simulink model "hcu_main_ADASwEPS"  (Simulink 8.2)
settings: Solver=FixedStepDiscrete  StartTime=0.0  StopTime=inf  FixedStep=0.001  RelTol=1e-3
PostLoadFcn:
  | , if any(exist('dsrtsu_mdlpostloadfcn', 'file') == [2, 3, 6]), try dsrtsu_mdlpostloadfcn('Execute', bdroot); catch fprintf('Error in PostLoadFcn (dsrtsu_mdlpostloadfcn) for model "%s":\n %s\n', bdroot, lasterr); end, end,
values from neighbouring files (symbols this model uses):
  C_TASK_1MS_S = (	C_TICK_TIME_S       )    [hcu_local_hdr.m]    (also in temp_ovrd_values.m = double(	0.001                  ))
  C_TICK_TIME_S = single(	0.005	    	)    [hcu_local_hdr.m]
  ENUM_EPSLFCSTATUS_ACTIVE = uint8(  2  )    [hcu_local_hdr.m]
  ENUM_EPSLFCSTATUS_TRANSITION = uint8(  3  )    [hcu_local_hdr.m]
  ENUM_EPSLKASTATUS_ACTIVE = uint8(  2  )    [hcu_local_hdr.m]
  ENUM_EPSMODEREQ_ANGLE = uint8(  1  )    [hcu_local_hdr.m]
  ENUM_EPSMODEREQ_INTERNAL = uint8(  0  )    [hcu_local_hdr.m]
  ENUM_EPSMODEREQ_TORQUE = uint8(  2  )    [hcu_local_hdr.m]
  ENUM_GEARPOSN_1ST = uint8(  1  )    [hcu_local_hdr.m]
  ENUM_GEARPOSN_2ND = uint8(  2  )    [hcu_local_hdr.m]
  ENUM_GEARPOSN_3RD = uint8(  3  )    [hcu_local_hdr.m]
  ENUM_GEARPOSN_4TH = uint8(  4  )    [hcu_local_hdr.m]
  ENUM_GEARPOSN_5TH = uint8(  5  )    [hcu_local_hdr.m]
  ENUM_GEARPOSN_6TH = uint8(  6  )    [hcu_local_hdr.m]
  ENUM_GEARPOSN_R = uint8(  7  )    [hcu_local_hdr.m]
  FALSE = boolean( 0 )    [hcu_local_hdr.m]
  TRUE = boolean( 1 )    [hcu_local_hdr.m]
undefined symbols (not defined in the file or in its folder): AISP_EPSCurrent_pct, AISP_TqASensorDelta_pct, AISP_TqBSensorDelta_pct, dHAL_IN, hal, INVALID_ABS1_TIMEOUT, INVALID_ABS2_TIMEOUT, INVALID_ABS3_TIMEOUT, INVALID_ABS4_TIMEOUT, INVALID_AC1_TIMEOUT, INVALID_ADASTORQ_REQ, INVALID_BCM1_TIMEOUT, INVALID_BCM2_TIMEOUT, INVALID_BOOSTER_VAC, INVALID_CSW1_TIMEOUT, INVALID_CUR_VEHDECE, INVALID_CURBRAKEDECE_REQ, INVALID_CURSTEERANG_REQ, INVALID_CURSTEERTQ_REQ, INVALID_ECM1_TIMEOUT, INVALID_ECM2_TIMEOUT, INVALID_ECM3_TIMEOUT, INVALID_ECM9_TIMEOUT, INVALID_ENG_TORQUE_FRICTIONAL, INVALID_ENG_TORQUE_INDICATED, INVALID_ENG_TORQUE_INDICATEDCOR, INVALID_ENG_TQ_MAX, INVALID_ENG_TQ_MIN, INVALID_EPAS2_TIMEOUT, INVALID_EPAS3_TIMEOUT, INVALID_EPB1_TIMEOUT, INVALID_EPS_BATTVOLT, INVALID_ESC_BATTVOLT, INVALID_GRADE, INVALID_HCU3_TIMEOUT, INVALID_HCU4_TIMEOUT, INVALID_HMI1_TIMEOUT, INVALID_HMI2_TIMEOUT, INVALID_LAT_ACC, INVALID_LONG_ACC, INVALID_MC_PRESSURE, INVALID_METER1_TIMEOUT, INVALID_METER3_TIMEOUT, INVALID_METER_VEHSPD, INVALID_ODO_METER, INVALID_OUTSIDE_TEMP, INVALID_PARKBRAKEBIND_STAT, INVALID_PEDALTQ_REQ, INVALID_SAS1_TIMEOUT, INVALID_SAS_ANGLE, INVALID_SHIFTER_POSN, INVALID_TCM1_TIMEOUT, INVALID_TCM2_TIMEOUT, INVALID_VCU1_TIMEOUT, INVALID_VCU2_TIMEOUT, INVALID_VEH_CRASH, INVALID_VEH_SPD, INVALID_WHEEL_SPD, INVALID_YAW_RATE, KHAL_MssgIdObj1_num ... (+8)
libraries: simulink x147, hcu_lib x38, rti1401lib_dio_type3 x4, rtimmsu_dsrtlib x3, app x1, rtiethernetudplib x1, rti1401lib_adc_type4 x1, rti1401lib_dac_type3 x1, inp x1, lidr x1, outp x1
(part 8 of 15)

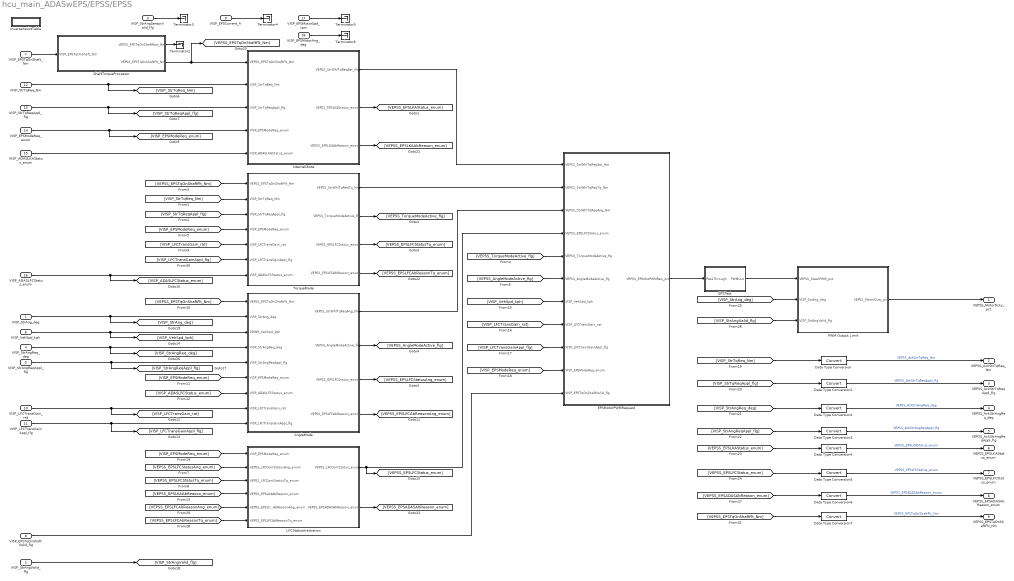
== system hcu_main_ADASwEPS/EPSS/EPSS ==
  VISP_StrAng_deg : Inport
  VISP_StrAngValid_flg : Inport  Port=2
  VISP_StrAngSensorValid_flg : Inport  Port=3
  VISP_StrAngReq_deg : Inport  Port=4
  VISP_StrAngReqAppl_flg : Inport  Port=5
  VISP_VehSpd_kph : Inport  Port=6
  VISP_EPSTqOnShaft_Nm : Inport  Port=7
  VISP_EPSTqOnShaftValid_flg : Inport  Port=8
  VISP_EPSCurrent_A : Inport  Port=9
  VISP_LFCTransGain_rat : Inport  Port=10
  VISP_LFCTransGainAppl_flg : Inport  Port=11
  VISP_StrTqReq_Nm : Inport  Port=12
  VISP_StrTqReqAppl_flg : Inport  Port=13
  VISP_EPSModeReq_enum : Inport  Port=14
  VISP_ADASLKAStatus_enum : Inport  Port=15
  VISP_ADASLFCStatus_enum : Inport  Port=16
  VISP_EPSMotorSpd_rpm : Inport  Port=17
  VISP_EPSMotorAng_deg : Inport  Port=18
  AngleMode : Subsystem
  Data Type Conversion{,1..7} (8 alike) : DataTypeConversion
  EPSMotorPWMRequest : Subsystem
  EPSTest : Subsystem
  InternalMode : Subsystem
  InverseAssistTable : Subsystem
  LFCStatusArbitration : Subsystem
  PWM Output Limit : Subsystem
  ShaftTorqueProcessor : Subsystem
  Terminator{2..6} (5 alike) : Terminator
  TorqueMode : Subsystem
  VEPSS_MotorDuty_pct : Outport
  VEPSS_AckStrTqReq_Nm : Outport  Port=2
  VEPSS_AckStrTqReqAppl_flg : Outport  Port=3
  VEPSS_AckStrAngReq_deg : Outport  Port=4
  VEPSS_AckStrAngReqAppl_flg : Outport  Port=5
  VEPSS_EPSLKAStatus_enum : Outport  Port=6
  VEPSS_EPSLFCStatus_enum : Outport  Port=7
  VEPSS_EPSADASAbReason_enum : Outport  Port=8
  VEPSS_EPSTqOnShaftFlt_Nm : Outport  Port=9
  wires:
  PWM Output Limit/1(VEPSS_MotorDuty_pct) -> VEPSS_MotorDuty_pct/1
  EPSMotorPWMRequest/1(VEPSS_EPSMotPWMReq_pct) -> EPSTest/1(PassThrough)
  EPSTest/1(PWMOut) -> PWM Output Limit/1(VEPSS_SteerPWM_pct)
  ShaftTorqueProcessor/2(VEPSS_EPSTqOnShaftFlt_Nm) -> [VEPSS_EPSTqOnShaftFlt_Nm], InternalMode/1(VEPSS_EPSTqOnShaftFlt_Nm)
  TorqueMode/1(VEPSS_StrWhlTqReqTq_Nm) -> EPSMotorPWMRequest/2(VEPSS_StrWhlTqReqTq_Nm)
  AngleMode/1(VEPSS_StrWhlTqReqAng_Nm) -> EPSMotorPWMRequest/3(VEPSS_StrWhlTqReqAng_Nm)
  InternalMode/1(VEPSS_StrWhlTqReqAst_Nm) -> EPSMotorPWMRequest/1(VEPSS_StrWhlTqReqAst_Nm)
  InternalMode/2(VEPSS_EPSLKAStatus_enum) -> [VEPSS_EPSLKAStatus_enum]
  TorqueMode/2(VEPSS_TorqueModeActive_flg) -> [VEPSS_TorqueModeActive_flg]
  TorqueMode/3(VEPSS_EPSLFCStatus_enum) -> [VEPSS_EPSLFCStatusTq_enum]
  AngleMode/2(VEPSS_AngleModeActive_flg) -> [VEPSS_AngleModeActive_flg]
  AngleMode/3(VEPSS_EPSLFCStatus_enum) -> [VEPSS_EPSLFCStatusAng_enum]
  [VEPSS_TorqueModeActive_flg] -> EPSMotorPWMRequest/5(VEPSS_TorqueModeActive_flg)
  [VEPSS_AngleModeActive_flg] -> EPSMotorPWMRequest/6(VEPSS_AngleModeActive_flg)
  LFCStatusArbitration/1(VEPSS_LFCContStatus_enum) -> EPSMotorPWMRequest/4(VEPSS_EPSLFCStatus_enum), [VEPSS_EPSLFCStatus_enum]
  [VEPSS_EPSLFCStatusTq_enum] -> LFCStatusArbitration/3(VEPSS_LFCContStatusTq_enum)
  [VEPSS_EPSLFCStatusAng_enum] -> LFCStatusArbitration/2(VEPSS_LFCContStatusAng_enum)
  ShaftTorqueProcessor/1(VEPSS_EPSTqOnShaftRaw_Nm) -> Terminator2/1
  VISP_EPSTqOnShaft_Nm/1 -> ShaftTorqueProcessor/1(VISP_EPSTqOnShaft_Nm)
  VISP_StrTqReqAppl_flg/1 -> [VISP_StrTqReqAppl_flg], InternalMode/3(VISP_StrTqReqAppl_flg)
  VISP_StrTqReq_Nm/1 -> [VISP_StrTqReq_Nm], InternalMode/2(VISP_StrTqReq_Nm)
  VISP_EPSModeReq_enum/1 -> [VISP_EPSModeReq_enum], InternalMode/4(VISP_EPSModeReq_enum)
  VISP_ADASLKAStatus_enum/1 -> InternalMode/5(VISP_ADASLKAStatus_enum)
  [VISP_StrTqReq_Nm] -> TorqueMode/2(VISP_StrTqReq_Nm)
  [VISP_StrTqReqAppl_flg] -> TorqueMode/3(VISP_StrTqReqAppl_flg)
  [VEPSS_EPSTqOnShaftFlt_Nm] -> TorqueMode/1(VEPSS_EPSTqOnShaftFlt_Nm)
  [VISP_EPSModeReq_enum] -> TorqueMode/4(VISP_EPSModeReq_enum)
  VISP_ADASLFCStatus_enum/1 -> [VISP_ADASLFCStatus_enum], TorqueMode/7(VISP_ADASLFCStatus_enum)
  VISP_StrAng_deg/1 -> [VISP_StrAng_deg], AngleMode/2(VISP_StrAng_deg)
  VISP_StrAngReq_deg/1 -> [VISP_StrAngReq_deg], AngleMode/4(VISP_StrAngReq_deg)
  VISP_StrAngReqAppl_flg/1 -> [VISP_StrAngReqAppl_flg], AngleMode/5(VISP_StrAngReqAppl_flg)
  [VEPSS_EPSTqOnShaftFlt_Nm] -> AngleMode/1(VEPSS_EPSTqOnShaftFlt_Nm)
  [VISP_EPSModeReq_enum] -> AngleMode/6(VISP_EPSModeReq_enum)
  [VISP_ADASLFCStatus_enum] -> AngleMode/7(VISP_ADASLFCStatus_enum)
  VISP_LFCTransGain_rat/1 -> [VISP_LFCTransGain_rat], AngleMode/8(VISP_LFCTransGain_rat)
  VISP_LFCTransGainAppl_flg/1 -> [VISP_LFCTransGainAppl_flg], AngleMode/9(VISP_LFCTransGainAppl_flg)
  [VISP_EPSModeReq_enum] -> LFCStatusArbitration/1(VISP_EPSModeReq_enum)
  VISP_VehSpd_kph/1 -> [VISP_VehSpd_kph], AngleMode/3(VDINR_VehSpd_kph)
  [VISP_VehSpd_kph] -> EPSMotorPWMRequest/7(VISP_VehSpd_kph)
  [VISP_LFCTransGain_rat] -> EPSMotorPWMRequest/8(VISP_LFCTransGain_rat)
  [VISP_LFCTransGainAppl_flg] -> EPSMotorPWMRequest/9(VISP_LFCTransGainAppl_flg)
  [VISP_EPSModeReq_enum] -> EPSMotorPWMRequest/10(VISP_EPSModeReq_enum)
  VISP_EPSTqOnShaftValid_flg/1 -> EPSMotorPWMRequest/11(VISP_EPSTqOnShaftValid_flg)
  VISP_StrAngValid_flg/1 -> [VISP_StrAngValid_flg]
  VISP_StrAngSensorValid_flg/1 -> Terminator3/1
  VISP_EPSCurrent_A/1 -> Terminator4/1
  VISP_EPSMotorSpd_rpm/1 -> Terminator5/1
  VISP_EPSMotorAng_deg/1 -> Terminator6/1
  [VISP_StrTqReqAppl_flg] -> Data Type Conversion1/1
  [VISP_StrAngReqAppl_flg] -> Data Type Conversion3/1
  [VEPSS_EPSLKAStatus_enum] -> Data Type Conversion4/1
  [VEPSS_EPSLFCStatus_enum] -> Data Type Conversion5/1
  Data Type Conversion/1 -> VEPSS_AckStrTqReq_Nm/1  "VEPSS_AckStrTqReq_Nm"
  Data Type Conversion1/1 -> VEPSS_AckStrTqReqAppl_flg/1  "VEPSS_AckStrTqReqAppl_flg"
  Data Type Conversion2/1 -> VEPSS_AckStrAngReq_deg/1  "VEPSS_AckStrAngReq_deg"
  Data Type Conversion3/1 -> VEPSS_AckStrAngReqAppl_flg/1  "VEPSS_AckStrAngReqAppl_flg"
  Data Type Conversion4/1 -> VEPSS_EPSLKAStatus_enum/1  "VEPSS_EPSLKAStatus_enum"
  Data Type Conversion5/1 -> VEPSS_EPSLFCStatus_enum/1  "VEPSS_EPSLFCStatus_enum"
  Data Type Conversion6/1 -> VEPSS_EPSADASAbReason_enum/1  "VEPSS_EPSADASAbReason_enum"
  [VISP_StrAng_deg] -> PWM Output Limit/2(VISP_StrAng_deg)
  [VISP_StrAngValid_flg] -> PWM Output Limit/3(VISP_StrAngValid_flg)
  InternalMode/3(VEPSS_EPSLKAAbReason_enum) -> [VEPSS_EPSLKAAbReason_enum]
  [VISP_LFCTransGain_rat] -> TorqueMode/5(VISP_LFCTransGain_rat)
  TorqueMode/4(VEPSS_EPSLFCAbReason_enum) -> [VEPSS_EPSLFCAbReasonTq_enum]
  AngleMode/4(VEPSS_EPSLFCAbReason_enum) -> [VEPSS_EPSLFCAbReasonAng_enum]
  [VEPSS_EPSLFCAbReasonAng_enum] -> LFCStatusArbitration/5(VEPSS_EPSLFCAbReasonAng_enum)
  [VEPSS_EPSLFCAbReasonTq_enum] -> LFCStatusArbitration/6(VEPSS_EPSLFCAbReasonTq_enum)
  LFCStatusArbitration/2(VEPSS_EPSADASAbReason_enum) -> [VEPSS_EPSADASAbReason_enum]
  [VEPSS_EPSADASAbReason_enum] -> Data Type Conversion6/1
  [VEPSS_EPSLKAAbReason_enum] -> LFCStatusArbitration/4(VEPSS_EPSLKAAbReason_enum)
  [VISP_StrTqReq_Nm] -> Data Type Conversion/1
  [VISP_StrAngReq_deg] -> Data Type Conversion2/1
  [VISP_LFCTransGainAppl_flg] -> TorqueMode/6(VISP_LFCTransGainAppl_flg)
  Data Type Conversion7/1 -> VEPSS_EPSTqOnShaftFlt_Nm/1  "VEPSS_EPSTqOnShaftFlt_Nm"
  [VEPSS_EPSTqOnShaftFlt_Nm] -> Data Type Conversion7/1

== system hcu_main_ADASwEPS/EPSS/model_info ==
  EmptySubsystem : Subsystem

== system hcu_main_ADASwEPS/ISP/AngleProcessing ==
  KISP_EPSZeroReset_flg : Inport
  VHAL_RelStrAng_deg : Inport  Port=2
  VHAL_VehSpd_kph : Inport  Port=3
  VHAL_YawRate_degps : Inport  Port=4
  VHAL_YawRateValid_flg : Inport  Port=5
  VHAL_LRRawWhlSpd_kph : Inport  Port=6
  VHAL_LRRawWhlSpdValid_flg : Inport  Port=7
  VHAL_RRRawWhlSpd_kph : Inport  Port=8
  VHAL_RRRawWhlSpdValid_flg : Inport  Port=9
  Abs : Abs
  Abs1 : Abs
  AbsAngCheckTime_s : Constant  Value=5
  Add : Sum  Inputs=+-
  Add1 : Sum  Inputs=+-
  KISP_AbsAngVehSpdthr_kph : Constant  Value=8
  KISP_AbsAngWhlSpdDifstr_kph : Constant  Value=0.5
  KISP_AbsAngYawRatethr_degps : Constant  Value=0.6
  Logical Operator : Logic  AllPortsSameDT=off  OutDataTypeStr=boolean
  Logical Operator1 : Logic  Operator=NOT  AllPortsSameDT=off  OutDataTypeStr=boolean
  Logical Operator2 : Logic  Inputs=6  AllPortsSameDT=off  OutDataTypeStr=boolean
  Logical Operator3 : Logic  Operator=OR  AllPortsSameDT=off  OutDataTypeStr=boolean
  Relational Operator : RelationalOperator  OutDataTypeStr=boolean
  Relational Operator1 : RelationalOperator  Operator=<=  OutDataTypeStr=boolean
  Relational Operator2 : RelationalOperator  OutDataTypeStr=boolean
  Relational Operator3 : RelationalOperator  Operator=<=  OutDataTypeStr=boolean
  Saturation : Saturate  UpperLimit=720  LowerLimit=-720
  Timer : Subsystem
  Triggered Absolute Angle Zero : Subsystem  TreatAsAtomicUnit=on
  Unit Delay : UnitDelay  SampleTime=-1
  VISP_StrAng_deg : Outport
  VISP_StrAngValid_flg : Outport  Port=2
  wires:
  VHAL_VehSpd_kph/1 -> Relational Operator/1
  KISP_AbsAngVehSpdthr_kph/1 -> Relational Operator/2
  VHAL_YawRate_degps/1 -> Abs/1
  Abs/1 -> Relational Operator1/1
  KISP_AbsAngYawRatethr_degps/1 -> Relational Operator1/2
  Relational Operator1/1 -> Timer/Enable
  Timer/1(Time_s) -> Relational Operator2/1
  AbsAngCheckTime_s/1 -> Relational Operator2/2
  VHAL_RRRawWhlSpd_kph/1 -> Add/2
  VHAL_LRRawWhlSpd_kph/1 -> Add/1
  Add/1 -> Abs1/1
  Abs1/1 -> Relational Operator3/1
  KISP_AbsAngWhlSpdDifstr_kph/1 -> Relational Operator3/2
  Relational Operator/1 -> Logical Operator2/1
  Relational Operator2/1 -> Logical Operator2/2
  VHAL_YawRateValid_flg/1 -> Logical Operator2/3
  VHAL_LRRawWhlSpdValid_flg/1 -> Logical Operator2/4
  Relational Operator3/1 -> Logical Operator2/5
  VHAL_RRRawWhlSpdValid_flg/1 -> Logical Operator2/6
  Logical Operator2/1 -> Logical Operator/1
  Unit Delay/1 -> Logical Operator1/1
  Triggered Absolute Angle Zero/2(Out2) -> VISP_StrAngValid_flg/1, Unit Delay/1  "VISP_StrAngValid_flg"
  Logical Operator1/1 -> Logical Operator/2
  Logical Operator/1 -> Logical Operator3/2
  VHAL_RelStrAng_deg/1 -> Add1/1, Triggered Absolute Angle Zero/1(In)
  Triggered Absolute Angle Zero/1(Out1) -> Add1/2
  Add1/1 -> Saturation/1
  Saturation/1 -> VISP_StrAng_deg/1  "VISP_StrAng_deg"
  Logical Operator3/1 -> Triggered Absolute Angle Zero/Trigger
  KISP_EPSZeroReset_flg/1 -> Logical Operator3/1

== system hcu_main_ADASwEPS/ISP/PassThrough ==
  VHAL_RelStrAng_deg : Inport
  VHAL_VehSpd_kph : Inport  Port=2
  VHAL_StrAngReqAppl_flg : Inport  Port=3
  VHAL_StrAngReq_deg : Inport  Port=4
  VHAL_LFCTransGainAppl_flg : Inport  Port=5
  VHAL_LFCTransGain_rat : Inport  Port=6
  VHAL_LatAccel_mps2 : Inport  Port=7
  VHAL_StrTqReqAppl_flg : Inport  Port=8
  VHAL_StrTqReq_Nm : Inport  Port=9
  VHAL_EPSModeReq_enum : Inport  Port=10
  VHAL_ADASLKAStatus_enum : Inport  Port=11
  VHAL_ADASLFCStatus_enum : Inport  Port=12
  VHAL_EPSMotorSpd_rpm : Inport  Port=13
  VHAL_EPSMotorAng_deg : Inport  Port=14
  Data Type Conversion{,1..12,14} (14 alike) : DataTypeConversion
  EPSDegTest : Subsystem
  SteerAngSensorValid : Constant  Value=TRUE
  StrAngCmdOvr : Constant  Value=FALSE
  StrAngCmdVal : Constant  Value=0
  Switch1 : Switch  Criteria=u2 ~= 0
  Switch2 : Switch  Criteria=u2 ~= 0
  VISP_StrAngSensorValid_flg : Outport
  VISP_StrAngReqAppl_flg : Outport  Port=2
  VISP_StrAngReq_deg : Outport  Port=3
  VISP_VehSpd_kph : Outport  Port=4
  VISP_RelStrAng_deg : Outport  Port=5
  VISP_LFCTransGainAppl_flg : Outport  Port=6
  VISP_LFCTransGain_rat : Outport  Port=7
  VISP_LatAccel_mps2 : Outport  Port=8
  VISP_StrTqReqAppl_flg : Outport  Port=9
  VISP_StrTqReq_Nm : Outport  Port=10
  VISP_EPSModeReq_enum : Outport  Port=11
  VISP_ADASLKAStatus_enum : Outport  Port=12
  VISP_ADASLFCStatus_enum : Outport  Port=13
  VISP_EPSMotorSpd_rpm : Outport  Port=14
  VISP_EPSMotorAng_deg : Outport  Port=15
  wires:
  SteerAngSensorValid/1 -> VISP_StrAngSensorValid_flg/1  "VISP_StrAngSensorValid_flg"
  VHAL_StrAngReqAppl_flg/1 -> Switch1/3
  Data Type Conversion/1 -> VISP_StrAngReq_deg/1  "VISP_StrAngReq_deg"
  Data Type Conversion1/1 -> VISP_StrAngReqAppl_flg/1  "VISP_StrAngReqAppl_flg"
  VHAL_VehSpd_kph/1 -> Data Type Conversion2/1
  Data Type Conversion2/1 -> VISP_VehSpd_kph/1  "VISP_VehSpd_kph"
  VHAL_RelStrAng_deg/1 -> Data Type Conversion3/1
  Data Type Conversion3/1 -> VISP_RelStrAng_deg/1  "VISP_RelStrAng_deg"
  StrAngCmdOvr/1 -> Switch1/1, Switch2/2, Switch1/2
  Switch1/1 -> Data Type Conversion1/1
  Switch2/1 -> Data Type Conversion/1
  StrAngCmdVal/1 -> EPSDegTest/1(PassThrough)
  EPSDegTest/1(DegOut) -> Switch2/1
  Data Type Conversion4/1 -> VISP_LFCTransGainAppl_flg/1  "VISP_LFCTransGainAppl_flg"
  Data Type Conversion5/1 -> VISP_LFCTransGain_rat/1  "VISP_LFCTransGain_rat"
  VHAL_LFCTransGainAppl_flg/1 -> Data Type Conversion4/1
  VHAL_LFCTransGain_rat/1 -> Data Type Conversion5/1
  VHAL_LatAccel_mps2/1 -> Data Type Conversion6/1
  Data Type Conversion6/1 -> VISP_LatAccel_mps2/1  "VISP_LatAccel_mps2"
  VHAL_StrTqReqAppl_flg/1 -> Data Type Conversion7/1
  Data Type Conversion7/1 -> VISP_StrTqReqAppl_flg/1  "VISP_StrTqReqAppl_flg"
  Data Type Conversion8/1 -> VISP_StrTqReq_Nm/1  "VISP_StrTqReq_Nm"
  VHAL_EPSMotorSpd_rpm/1 -> Data Type Conversion9/1
  Data Type Conversion9/1 -> VISP_EPSMotorSpd_rpm/1  "VISP_EPSMotorSpd_rpm"
  VHAL_EPSMotorAng_deg/1 -> Data Type Conversion10/1
  Data Type Conversion10/1 -> VISP_EPSMotorAng_deg/1  "VISP_EPSMotorAng_deg"
  VHAL_EPSModeReq_enum/1 -> Data Type Conversion11/1
  Data Type Conversion11/1 -> VISP_EPSModeReq_enum/1  "VISP_EPSModeReq_enum"
  VHAL_ADASLKAStatus_enum/1 -> Data Type Conversion12/1
  Data Type Conversion12/1 -> VISP_ADASLKAStatus_enum/1  "VISP_ADASLKAStatus_enum"
  VHAL_ADASLFCStatus_enum/1 -> Data Type Conversion14/1
  Data Type Conversion14/1 -> VISP_ADASLFCStatus_enum/1  "VISP_ADASLFCStatus_enum"
  VHAL_StrAngReq_deg/1 -> Switch2/3
  VHAL_StrTqReq_Nm/1 -> Data Type Conversion8/1

== system hcu_main_ADASwEPS/ISP/TqProcessing ==
  VHAL_TqSensorADuty_pct : Inport
  VHAL_TqSensorBDuty_pct : Inport  Port=2
  KISP_EPSZeroReset_flg : Inport  Port=3
  Add : Sum
  Gain : Gain  Gain=1/2
  LowPassFilter : Subsystem
  MISP_TqAOnShaft_Nm : Lookup  InputValues=AISP_TqASensorDelta_pct  Table=MISP_TqAOnShaft_Nm  LookUpMeth=Interpolation-Use End Values
      settings: AttributesFormatString="Input=\"%<InputValues>\"\\nOutput=\"%<Table>\""
  MISP_TqBOnShaft_Nm : Lookup  InputValues=AISP_TqBSensorDelta_pct  Table=MISP_TqBOnShaft_Nm  LookUpMeth=Interpolation-Use End Values
      settings: AttributesFormatString="Input=\"%<InputValues>\"\\nOutput=\"%<Table>\""
  Terminator5 : Terminator
  Terminator6 : Terminator
  TorqueValid : Subsystem
  TqSensorAZero : Subsystem
  TqSensorBZero : Subsystem
  TqSensorFlac_pct : Constant  Value=0.1
  VISP_EPSTqOnShaft_Nm : Outport
  VISP_EPSTqOnShaftValid_flg : Outport  Port=2
  wires:
  Gain/1 -> LowPassFilter/1(Raw)
  TqSensorBZero/2(delta) -> MISP_TqBOnShaft_Nm/1
  Add/1 -> Gain/1
  TqSensorAZero/2(delta) -> MISP_TqAOnShaft_Nm/1
  TqSensorAZero/1(zero) -> Terminator5/1
  TqSensorBZero/1(zero) -> Terminator6/1
  TqSensorFlac_pct/1 -> TqSensorBZero/2(TqSensorFlac_pct), TqSensorAZero/2(TqSensorFlac_pct)
  KISP_EPSZeroReset_flg/1 -> TqSensorBZero/3(KISP_EPSZeroReset_flg), TqSensorAZero/3(KISP_EPSZeroReset_flg)
  MISP_TqAOnShaft_Nm/1 -> TorqueValid/1(TqA), Add/1
  TorqueValid/1(TqValid_flg) -> VISP_EPSTqOnShaftValid_flg/1  "VISP_EPSTqOnShaftValid_flg"
  MISP_TqBOnShaft_Nm/1 -> TorqueValid/2(TqB), Add/2
  VHAL_TqSensorADuty_pct/1 -> TqSensorAZero/1(VHAL_TqSensorADuty_pct)
  VHAL_TqSensorBDuty_pct/1 -> TqSensorBZero/1(VHAL_TqSensorBDuty_pct)
  LowPassFilter/1(Out) -> VISP_EPSTqOnShaft_Nm/1  "VISP_EPSTqOnShaft_Nm"

== system hcu_main_ADASwEPS/OSP/OSP ==
  BISP_outputs : Inport
  BEPSS_outputs : Inport  Port=2
  Bus Creator5 : BusCreator  Inputs=24
  Bus Selector : BusSelector  OutputSignals=VEPSS_EPSTqOnShaftFlt_Nm
  Bus Selector1 : BusSelector  OutputSignals=VEPSS_MotorDuty_pct,VEPSS_AckStrAngReq_deg,VEPSS_AckStrTqReq_Nm,VEPSS_AckStrAngReqAppl_flg,VEPSS_AckStrTqReqAppl_flg,VEPSS_EPSLKAStatus_enum,VEPSS_EPSLFCStatus_enum,VEPSS_EPSADASAbReason_enum
  Bus Selector2 : BusSelector  OutputSignals=VISP_EPSTqOnShaftValid_flg
  Bus Selector3 : BusSelector  OutputSignals=VISP_StrAng_deg,VISP_RelStrAng_deg,VISP_StrAngValid_flg,VISP_StrAngSensorValid_flg
  CheckSum Calculation : Subsystem  TreatAsAtomicUnit=on
  CheckSum Calculation1 : Subsystem  TreatAsAtomicUnit=on
  CheckSum Calculation2 : Subsystem  TreatAsAtomicUnit=on
  Constant : Constant  Value=15  OutDataTypeStr=uint8
  Constant1 : Constant  Value=15  OutDataTypeStr=uint8
  Constant2 : Constant  Value=15  OutDataTypeStr=uint8
  Constant4 : Constant  Value=TRUE
  Constant5 : Constant  Value=0.01
  Constant6 : Constant  Value=0.01
  Constant7 : Constant  Value=0.01
  Data Type Conversion{1..2,7,11,17,23..24,33} (8 alike) : DataTypeConversion  OutDataTypeStr=double
  Data Type Conversion{4..5,10,16,18,25..26} (7 alike) : DataTypeConversion  OutDataTypeStr=boolean
  Data Type Conversion{3,15,19..22,27,29..30} (9 alike) : DataTypeConversion  OutDataTypeStr=uint8
  EPSBattVolt : Constant  Value=12
  EpasFailed : Constant  Value=FALSE
  Function Call Generator EPAS2 : Stateflow chart  TreatAsAtomicUnit=on
  Function Call Generator EPAS3 : Stateflow chart  TreatAsAtomicUnit=on
  Function Call Generator SAS1 : Stateflow chart  TreatAsAtomicUnit=on
  RollCnt : Subsystem
  RollCnt1 : Subsystem
  RollCnt2 : Subsystem
  ZeroPower : Constant  Value=0
  BOSP_outputs : Outport
  wires:
  Bus Creator5/1 -> BOSP_outputs/1
  EpasFailed/1 -> Data Type Conversion10/1
  Data Type Conversion10/1 -> Bus Creator5/9  "VOSP_EpasFailed_flg"
  Data Type Conversion11/1 -> Bus Creator5/8  "VOSP_ElectPWRConsumpt_A"
  Data Type Conversion1/1 -> Bus Creator5/14  "VOSP_MotorDuty_pct"
  BEPSS_outputs/1 -> [BEPSS_outputs], CheckSum Calculation2/1(BEPSS_outputs), Bus Selector1/1
  Bus Selector1/1 -> Data Type Conversion1/1  "<VEPSS_MotorDuty_pct>"
  BISP_outputs/1 -> Bus Selector2/1, CheckSum Calculation/1(BISP_outputs), CheckSum Calculation1/2(BISP_outputs), Bus Selector3/1
  Bus Selector3/1 -> Data Type Conversion2/1  "<VISP_StrAng_deg>"
  Data Type Conversion2/1 -> Bus Creator5/1  "VOSP_StrAng_deg"
  Data Type Conversion4/1 -> Bus Creator5/3  "VOSP_StrAngCal_flg"
  Data Type Conversion5/1 -> Bus Creator5/4  "VOSP_RelStrAngValid_flg"
  Bus Selector3/2 -> Data Type Conversion7/1  "<VISP_RelStrAng_deg>"
  Data Type Conversion7/1 -> Bus Creator5/2  "VOSP_RelStrAng_deg"
  Bus Selector3/4 -> Data Type Conversion16/1  "<VISP_StrAngSensorValid_flg>"
  Data Type Conversion16/1 -> Bus Creator5/5  "VOSP_StrAngSensorValid_flg"
  Bus Selector/1 -> Data Type Conversion17/1  "<VEPSS_EPSTqOnShaftFlt_Nm>"
  Data Type Conversion17/1 -> Bus Creator5/6  "VOSP_StrTq_Nm"
  Bus Selector2/1 -> Data Type Conversion18/1  "<VISP_EPSTqOnShaftValid_flg>"
  Data Type Conversion18/1 -> Bus Creator5/7  "VOSP_StrTqValid_flg"
  ZeroPower/1 -> Data Type Conversion11/1
  Constant/1 -> RollCnt/1(max)
  RollCnt/1(out) -> Data Type Conversion15/1, CheckSum Calculation/2(LifeCount)
  Constant1/1 -> RollCnt1/1(max)
  RollCnt1/1(out) -> Data Type Conversion19/1, CheckSum Calculation1/3(LifeCount)
  Data Type Conversion15/1 -> Bus Creator5/11  "VOSP_SAS1RollCnt_cnt"
  Data Type Conversion19/1 -> Bus Creator5/13  "VOSP_EPAS2RollCnt_cnt"
  Constant2/1 -> RollCnt2/1(max)
  RollCnt2/1(out) -> CheckSum Calculation2/2(LifeCount), Data Type Conversion20/1
  Data Type Conversion20/1 -> Bus Creator5/24  "VOSP_EPAS3RollCnt_cnt"
  CheckSum Calculation/1(VOSP_SAS1CalcChecksum_raw8) -> Data Type Conversion21/1
  Data Type Conversion21/1 -> Bus Creator5/10  "VOSP_SAS1CalcChecksum_raw8"
  Data Type Conversion22/1 -> Bus Creator5/12  "VOSP_EPAS2CalcChecksum_raw8"
  CheckSum Calculation1/1(VOSP_EPAS2CalcChecksum_raw8) -> Data Type Conversion22/1
  Bus Selector1/2 -> Data Type Conversion23/1  "<VEPSS_AckStrAngReq_deg>"
  Data Type Conversion23/1 -> Bus Creator5/15  "VOSP_AckStrAngReq_deg"
  Bus Selector1/3 -> Data Type Conversion24/1  "<VEPSS_AckStrTqReq_Nm>"
  Data Type Conversion24/1 -> Bus Creator5/16  "VOSP_AckStrTqReq_Nm"
  Bus Selector1/4 -> Data Type Conversion25/1  "<VEPSS_AckStrAngReqAppl_flg>"
  Data Type Conversion25/1 -> Bus Creator5/17  "VOSP_AckStrAngReqAppl_flg"
  Data Type Conversion26/1 -> Bus Creator5/18  "VOSP_AckStrTqReqAppl_flg"
  Bus Selector1/5 -> Data Type Conversion26/1  "<VEPSS_AckStrTqReqAppl_flg>"
  Bus Selector1/6 -> Data Type Conversion27/1  "<VEPSS_EPSLKAStatus_enum>"
  Data Type Conversion27/1 -> Bus Creator5/19  "VOSP_EPSLKAStatus_enum"
  Data Type Conversion29/1 -> Bus Creator5/21  "VOSP_EPSADASAbReason_enum"
  Bus Selector1/8 -> Data Type Conversion29/1  "<VEPSS_EPSADASAbReason_enum>"
  Data Type Conversion30/1 -> Bus Creator5/20  "VOSP_EPSLFCStatus_enum"
  Bus Selector1/7 -> Data Type Conversion30/1  "<VEPSS_EPSLFCStatus_enum>"
  Data Type Conversion33/1 -> Bus Creator5/22  "VOSP_EPSBattVolt_V"
  EPSBattVolt/1 -> Data Type Conversion33/1
  Bus Selector3/3 -> Data Type Conversion4/1  "<VISP_StrAngValid_flg>"
  Constant4/1 -> Data Type Conversion5/1
  Constant5/1 -> Function Call Generator SAS1/1(SampleTime_S)
  Function Call Generator SAS1/1(FunCall()) -> RollCnt/Trigger
  Constant6/1 -> Function Call Generator EPAS2/1(SampleTime_S)
  Function Call Generator EPAS2/1(FunCall()) -> RollCnt1/Trigger
  Constant7/1 -> Function Call Generator EPAS3/1(SampleTime_S)
  Function Call Generator EPAS3/1(FunCall()) -> RollCnt2/Trigger
  CheckSum Calculation2/1(VOSP_EPAS3CalcChecksum_raw8) -> Data Type Conversion3/1
  Data Type Conversion3/1 -> Bus Creator5/23  "VOSP_EPAS3CalcChecksum_raw8"
  [BEPSS_outputs] -> Bus Selector/1
  [BEPSS_outputs] -> CheckSum Calculation1/1(BEPSS_outputs)

== system hcu_main_ADASwEPS/RTI Data/RTI Data Store ==
  RTI Data Store : Subsystem  mask(RTI_DATA_STORE){}
      mask help:
      | RTI Data Store Block. This block is used by RTI to store internal model dependent data. Deleting this block will result in data loss.
      |
      | NEVER DELETE, COPY, OR MODIFY THIS BLOCK!
      mask Help:
      | RTI Data Store Block. This block is used by RTI to store internal model dependent data. Deleting this block will result in data loss.
      | 
      | NEVER DELETE, COPY, OR MODIFY THIS BLOCK!
      mask Display: text(0.5, 0.5, ' ', 'HorizontalAlignment', 'center');

== system hcu_main_ADASwEPS/RTICANMM ControllerSetup/ModelClose ==

== system hcu_main_ADASwEPS/RTICANMM ControllerSetup1/ModelClose ==

== system hcu_main_ADASwEPS/RTICANMM GeneralSetup/ModelClose ==

== system hcu_main_ADASwEPS/Triggering2CAN1/ADAS4 ==
  ADAS4_Kickout : Constant  Value=0
  buscreator : BusCreator  Inputs=1
  dt_ADAS4_Kickout : DataTypeConversion  RndMeth=Zero
  out : Outport
  wires:
  buscreator/1 -> out/1  "ADAS4"
  ADAS4_Kickout/1 -> dt_ADAS4_Kickout/1
  dt_ADAS4_Kickout/1 -> buscreator/1  "ADAS4_Kickout"

== system hcu_main_ADASwEPS/Triggering2CAN1/ADAS5 ==
  ADAS5_Kickout : Constant  Value=0
  buscreator : BusCreator  Inputs=1
  dt_ADAS5_Kickout : DataTypeConversion  RndMeth=Zero
  out : Outport
  wires:
  buscreator/1 -> out/1  "ADAS5"
  ADAS5_Kickout/1 -> dt_ADAS5_Kickout/1
  dt_ADAS5_Kickout/1 -> buscreator/1  "ADAS5_Kickout"

== system hcu_main_ADASwEPS/User2CAN1_/ADAS1 ==
  BOUTP_outputs : Inport  OutDataTypeStr=Bus: BOUTP_outputs
  ADAS1_Checksum : Ground
  Bus Selector : BusSelector  OutputSignals=VOUTP_ADAS1RollCnt_cnt,VOUTP_StrTqAppl_flg,VOUTP_StrAngAppl_flg,VOUTP_LFCTransGainAppl_flg,VOUTP_EPSModeReq_enum,VOUTP_ADASLKAStatus_enum,VOUTP_ADASLFCStatus_enum,VOUTP_StrTqReq_Nm,VOUTP_LFCTransGain_rat,VOUTP_StrAngReq_deg
  Data Type Conversion{1..10} (10 alike) : DataTypeConversion
  buscreator : BusCreator  Inputs=11
  out : Outport
  wires:
  buscreator/1 -> out/1  "ADAS1"
  ADAS1_Checksum/1 -> buscreator/1  "ADAS1_Checksum"
  Data Type Conversion2/1 -> buscreator/2  "ADAS1_LifeCount"
  Data Type Conversion1/1 -> buscreator/3  "ADAS_StrTqReq_A"
  Data Type Conversion3/1 -> buscreator/4  "ADAS_StrAngReq_A"
  Data Type Conversion5/1 -> buscreator/5  "ADAS_LFCTranGain_A"
  Data Type Conversion4/1 -> buscreator/6  "ADAS_EPSMode"
  Data Type Conversion6/1 -> buscreator/7  "ADAS_LKAStatus"
  Data Type Conversion8/1 -> buscreator/8  "ADAS_LFCStatus"
  Data Type Conversion7/1 -> buscreator/9  "ADAS_StrTqReq"
  Data Type Conversion9/1 -> buscreator/10  "ADAS_LFCTransGain"
  Data Type Conversion10/1 -> buscreator/11  "ADAS_StrAngReq"
  BOUTP_outputs/1 -> Bus Selector/1
  Bus Selector/2 -> Data Type Conversion1/1  "<VOUTP_StrTqAppl_flg>"
  Bus Selector/1 -> Data Type Conversion2/1  "<VOUTP_ADAS1RollCnt_cnt>"
  Bus Selector/3 -> Data Type Conversion3/1  "<VOUTP_StrAngAppl_flg>"
  Bus Selector/4 -> Data Type Conversion5/1  "<VOUTP_LFCTransGainAppl_flg>"
  Bus Selector/5 -> Data Type Conversion4/1  "<VOUTP_EPSModeReq_enum>"
  Bus Selector/6 -> Data Type Conversion6/1  "<VOUTP_ADASLKAStatus_enum>"
  Bus Selector/7 -> Data Type Conversion8/1  "<VOUTP_ADASLFCStatus_enum>"
  Bus Selector/8 -> Data Type Conversion7/1  "<VOUTP_StrTqReq_Nm>"
  Bus Selector/9 -> Data Type Conversion9/1  "<VOUTP_LFCTransGain_rat>"
  Bus Selector/10 -> Data Type Conversion10/1  "<VOUTP_StrAngReq_deg>"

== system hcu_main_ADASwEPS/User2CAN1_/ADAS2 ==
  BOUTP_outputs : Inport  OutDataTypeStr=Bus: BOUTP_outputs
  ADAS2_Checksum : Ground
  Bus Selector : BusSelector  OutputSignals=VOUTP_ADAS2RollCnt_cnt,VOUTP_VirtualGearRatio_enum,VOUTP_ADASACCStatus_enum,VOUTP_BrakeHapticReq_flg,VOUTP_VehHoldReq_flg,VOUTP_BrakePrefillReqAppl_flg,VOUTP_BrakePrefillReq_flg,VOUTP_AEBReqAppl_flg,VOUTP_AEBReq_flg,VOUTP_DecReq_mps2,VOUTP_ForceIdleAppl_flg,VOUTP_DecReqAppl_flg,VOUTP_PTTqReqAppl_flg,VOUTP_ForceIdle_flg,VOUTP_PTTqReq_Nm
  Data Type Conversion{1..11,13..16} (15 alike) : DataTypeConversion
  buscreator : BusCreator  Inputs=16
  out : Outport
  wires:
  buscreator/1 -> out/1  "ADAS2"
  ADAS2_Checksum/1 -> buscreator/1  "ADAS2_Checksum"
  Data Type Conversion2/1 -> buscreator/2  "ADAS2_LifeCount"
  Data Type Conversion1/1 -> buscreator/3  "ADAS_VirtualGear"
  Data Type Conversion3/1 -> buscreator/4  "ADAS_ACCStatus"
  Data Type Conversion5/1 -> buscreator/5  "ADAS_BHapticReq"
  Data Type Conversion4/1 -> buscreator/6  "ADAS_VehHoldReq"
  Data Type Conversion6/1 -> buscreator/7  "ADAS_BPrefillReq_A"
  Data Type Conversion8/1 -> buscreator/8  "ADAS_BPrefillReq"
  Data Type Conversion7/1 -> buscreator/9  "ADAS_AEBReq_A"
  Data Type Conversion9/1 -> buscreator/10  "ADAS_AEBReq"
  Data Type Conversion10/1 -> buscreator/11  "ADAS_DecReq"
  Data Type Conversion13/1 -> buscreator/12  "ADAS_ForceIdle_A"
  Data Type Conversion11/1 -> buscreator/13  "ADAS_DecReq_A"
  Data Type Conversion14/1 -> buscreator/14  "ADAS_PTTqReq_A"
  Data Type Conversion16/1 -> buscreator/15  "ADAS_ForceIdle"
  Data Type Conversion15/1 -> buscreator/16  "ADAS_PTTqReq"
  BOUTP_outputs/1 -> Bus Selector/1
  Bus Selector/1 -> Data Type Conversion2/1  "<VOUTP_ADAS2RollCnt_cnt>"
  Bus Selector/2 -> Data Type Conversion1/1  "<VOUTP_VirtualGearRatio_enum>"
  Bus Selector/3 -> Data Type Conversion3/1  "<VOUTP_ADASACCStatus_enum>"
  Bus Selector/4 -> Data Type Conversion5/1  "<VOUTP_BrakeHapticReq_flg>"
  Bus Selector/5 -> Data Type Conversion4/1  "<VOUTP_VehHoldReq_flg>"
  Bus Selector/6 -> Data Type Conversion6/1  "<VOUTP_BrakePrefillReqAppl_flg>"
  Bus Selector/7 -> Data Type Conversion8/1  "<VOUTP_BrakePrefillReq_flg>"
  Bus Selector/8 -> Data Type Conversion7/1  "<VOUTP_AEBReqAppl_flg>"
  Bus Selector/9 -> Data Type Conversion9/1  "<VOUTP_AEBReq_flg>"
  Bus Selector/10 -> Data Type Conversion10/1  "<VOUTP_DecReq_mps2>"
  Bus Selector/11 -> Data Type Conversion13/1  "<VOUTP_ForceIdleAppl_flg>"
  Bus Selector/12 -> Data Type Conversion11/1  "<VOUTP_DecReqAppl_flg>"
  Bus Selector/13 -> Data Type Conversion14/1  "<VOUTP_PTTqReqAppl_flg>"
  Bus Selector/14 -> Data Type Conversion16/1  "<VOUTP_ForceIdle_flg>"
  Bus Selector/15 -> Data Type Conversion15/1  "<VOUTP_PTTqReq_Nm>"

== system hcu_main_ADASwEPS/User2CAN1_/ADAS3 ==
  BOUTP_outputs : Inport  OutDataTypeStr=Bus: BOUTP_outputs
  ADAS3_Checksum : Ground
  Bus Selector : BusSelector  OutputSignals=VOUTP_ADAS3RollCnt_cnt,VOUTP_ShiftPosnReqAppl_flg,VOUTP_ShiftPosnReq_enum,VOUTP_VehSpdLimAppl_flg,VOUTP_GearPosnReqAppl_flg,VOUTP_GearPosnReq_enum,VOUTP_VehSpdLim_kph
  Data Type Conversion{7,9..11,13..14,16} (7 alike) : DataTypeConversion
  buscreator : BusCreator  Inputs=8
  out : Outport
  wires:
  buscreator/1 -> out/1  "ADAS3"
  ADAS3_Checksum/1 -> buscreator/1  "ADAS3_Checksum"
  Data Type Conversion7/1 -> buscreator/2  "ADAS3_LifeCount"
  Data Type Conversion9/1 -> buscreator/3  "ADAS_ShftPosnReq_A"
  Data Type Conversion10/1 -> buscreator/4  "ADAS_ShftPosnReq"
  Data Type Conversion13/1 -> buscreator/5  "ADAS_VehSpdLim_A"
  Data Type Conversion11/1 -> buscreator/6  "ADAS_GearPosnReq_A"
  Data Type Conversion14/1 -> buscreator/7  "ADAS_GearPosnReq"
  Data Type Conversion16/1 -> buscreator/8  "ADAS_VehSpdLim"
  BOUTP_outputs/1 -> Bus Selector/1
  Bus Selector/3 -> Data Type Conversion10/1  "<VOUTP_ShiftPosnReq_enum>"
  Bus Selector/4 -> Data Type Conversion13/1  "<VOUTP_VehSpdLimAppl_flg>"
  Bus Selector/2 -> Data Type Conversion9/1  "<VOUTP_ShiftPosnReqAppl_flg>"
  Bus Selector/5 -> Data Type Conversion11/1  "<VOUTP_GearPosnReqAppl_flg>"
  Bus Selector/1 -> Data Type Conversion7/1  "<VOUTP_ADAS3RollCnt_cnt>"
  Bus Selector/6 -> Data Type Conversion14/1  "<VOUTP_GearPosnReq_enum>"
  Bus Selector/7 -> Data Type Conversion16/1  "<VOUTP_VehSpdLim_kph>"

== system hcu_main_ADASwEPS/User2CAN1_/ADAS4 ==
  BOUTP_outputs : Inport  OutDataTypeStr=Bus: BOUTP_outputs
  Bus Selector : BusSelector  OutputSignals=VOUTP_ADASMILReq_flg,VOUTP_FaultWarningReq_flg,VOUTP_ForceLowBeam_flg,VOUTP_ADASFunOffSoundReq_flg,VOUTP_ADASFunOnSoundReq_flg,VOUTP_HazardWarningReq_flg,VOUTP_LFCHMIStatus_enum,VOUTP_LKAHMIStatus_enum,VOUTP_LFCWarningReq_flg,VOUTP_IGSAWarningReq_flg,VOUTP_AEBWarningReq_flg,VOUTP_ACCWarningReq_flg,VOUTP_FCWWarningReq_flg
  Data Type Conversion{1..30} (30 alike) : DataTypeConversion
  Ground{,1..9,12..16,19,21} (17 alike) : Ground
  buscreator : BusCreator  Inputs=30
  out : Outport
  wires:
  buscreator/1 -> out/1  "ADAS4"
  Data Type Conversion7/1 -> buscreator/1  "ADAS_MIL"
  Data Type Conversion9/1 -> buscreator/2  "ADASFaultWarnReq"
  Data Type Conversion10/1 -> buscreator/3  "ForceLowBeam"
  Data Type Conversion13/1 -> buscreator/6  "LeftTurnLightReq"
  Data Type Conversion11/1 -> buscreator/7  "RightTurnLightReq"
  Data Type Conversion14/1 -> buscreator/8  "HazardWarningReq"
  Data Type Conversion16/1 -> buscreator/9  "HapticWarningReq"
  Data Type Conversion6/1 -> buscreator/10  "APSEnable"
  Data Type Conversion8/1 -> buscreator/11  "PilotMode"
  Data Type Conversion1/1 -> buscreator/12  "IGSAStatus"
  Data Type Conversion3/1 -> buscreator/13  "LFCMode"
  Data Type Conversion2/1 -> buscreator/14  "MAPPStatus"
  Data Type Conversion4/1 -> buscreator/15  "MAPAStatus"
  Data Type Conversion5/1 -> buscreator/16  "LCSStatus"
  Data Type Conversion20/1 -> buscreator/17  "LFCStatus"
  Data Type Conversion21/1 -> buscreator/18  "LKAStatus"
  Data Type Conversion12/1 -> buscreator/19  "ACCStatus"
  Data Type Conversion17/1 -> buscreator/20  "FCWStatus"
  Data Type Conversion15/1 -> buscreator/21  "AEBStatus"
  Data Type Conversion18/1 -> buscreator/22  "MAPPHMIWarningReq"
  Data Type Conversion19/1 -> buscreator/23  "MAPAHMIWarningReq"
  Data Type Conversion27/1 -> buscreator/24  "LCSHMIWarningReq"
  Data Type Conversion28/1 -> buscreator/25  "LFCHMIWarningReq"
  Data Type Conversion22/1 -> buscreator/26  "LKAHMIWarningReq"
  Data Type Conversion24/1 -> buscreator/27  "IGSAHMIWarningReq"
  Data Type Conversion23/1 -> buscreator/28  "AEBHMIWarningReq"
  Data Type Conversion25/1 -> buscreator/29  "ACCHMIWarningReq"
  Data Type Conversion26/1 -> buscreator/30  "FCWHMIWarningReq"
  BOUTP_outputs/1 -> Bus Selector/1
  Bus Selector/1 -> Data Type Conversion7/1  "<VOUTP_ADASMILReq_flg>"
  Bus Selector/2 -> Data Type Conversion9/1  "<VOUTP_FaultWarningReq_flg>"
  Bus Selector/3 -> Data Type Conversion10/1  "<VOUTP_ForceLowBeam_flg>"
  Bus Selector/6 -> Data Type Conversion14/1  "<VOUTP_HazardWarningReq_flg>"
  Bus Selector/10 -> Data Type Conversion24/1  "<VOUTP_IGSAWarningReq_flg>"
  Bus Selector/11 -> Data Type Conversion23/1  "<VOUTP_AEBWarningReq_flg>"
  Bus Selector/12 -> Data Type Conversion25/1  "<VOUTP_ACCWarningReq_flg>"
  Bus Selector/13 -> Data Type Conversion26/1  "<VOUTP_FCWWarningReq_flg>"
  Ground/1 -> Data Type Conversion13/1
  Ground1/1 -> Data Type Conversion11/1
  Ground2/1 -> Data Type Conversion16/1
  Ground3/1 -> Data Type Conversion6/1
  Ground4/1 -> Data Type Conversion8/1
  Ground5/1 -> Data Type Conversion1/1
  Ground6/1 -> Data Type Conversion3/1
  Ground7/1 -> Data Type Conversion2/1
  Ground8/1 -> Data Type Conversion4/1
  Ground9/1 -> Data Type Conversion5/1
  Bus Selector/7 -> Data Type Conversion20/1  "<VOUTP_LFCHMIStatus_enum>"
  Bus Selector/8 -> Data Type Conversion21/1  "<VOUTP_LKAHMIStatus_enum>"
  Ground14/1 -> Data Type Conversion12/1
  Ground15/1 -> Data Type Conversion17/1
  Ground16/1 -> Data Type Conversion15/1
  Ground12/1 -> Data Type Conversion18/1
  Ground13/1 -> Data Type Conversion19/1
  Ground19/1 -> Data Type Conversion27/1
  Bus Selector/9 -> Data Type Conversion28/1  "<VOUTP_LFCWarningReq_flg>"
  Ground21/1 -> Data Type Conversion22/1
  Data Type Conversion29/1 -> buscreator/4  "OffSoundReq"
  Data Type Conversion30/1 -> buscreator/5  "OnSoundReq"
  Bus Selector/4 -> Data Type Conversion29/1  "<VOUTP_ADASFunOffSoundReq_flg>"
  Bus Selector/5 -> Data Type Conversion30/1  "<VOUTP_ADASFunOnSoundReq_flg>"

== system hcu_main_ADASwEPS/User2CAN1_/ADAS5 ==
  BOUTP_outputs : Inport  OutDataTypeStr=Bus: BOUTP_outputs
  Bus Selector : BusSelector  OutputSignals=VOUTP_ADASFaultMode_enum,VOUTP_NumberOfTargets_num,VOUTP_RightLaneLampMode_enum,VOUTP_LeftLaneLampMode_enum,VOUTP_ACCSetTimeGapTmp_enum,VOUTP_ACCSetTimeGap_enum,VOUTP_ACCSetSpeed_kph
  Data Type Conversion{1..11} (11 alike) : DataTypeConversion
  Ground{2..5} (4 alike) : Ground
  buscreator : BusCreator  Inputs=11
  out : Outport
  wires:
  buscreator/1 -> out/1  "ADAS5"
  Data Type Conversion7/1 -> buscreator/1  "ADAS_FaultMode"
  Data Type Conversion1/1 -> buscreator/3  "ADAS_LaneModeR"
  Data Type Conversion2/1 -> buscreator/4  "ADAS_LaneModeL"
  Data Type Conversion3/1 -> buscreator/5  "SeleTimeGapLvl"
  Data Type Conversion4/1 -> buscreator/6  "SetTimeGapLvl"
  Data Type Conversion5/1 -> buscreator/7  "IGSASetSpeed"
  Data Type Conversion6/1 -> buscreator/8  "ACCSetSpeed"
  Data Type Conversion8/1 -> buscreator/9  "SetVehTimeGap"
  Data Type Conversion9/1 -> buscreator/10  "LeadVehTimeGap"
  Data Type Conversion10/1 -> buscreator/11  "TargetType"
  BOUTP_outputs/1 -> Bus Selector/1
  Bus Selector/1 -> Data Type Conversion7/1  "<VOUTP_ADASFaultMode_enum>"
  Bus Selector/5 -> Data Type Conversion3/1  "<VOUTP_ACCSetTimeGapTmp_enum>"
  Bus Selector/6 -> Data Type Conversion4/1  "<VOUTP_ACCSetTimeGap_enum>"
  Bus Selector/7 -> Data Type Conversion6/1  "<VOUTP_ACCSetSpeed_kph>"
  Bus Selector/3 -> Data Type Conversion1/1  "<VOUTP_RightLaneLampMode_enum>"
  Bus Selector/4 -> Data Type Conversion2/1  "<VOUTP_LeftLaneLampMode_enum>"
  Ground2/1 -> Data Type Conversion5/1
  Ground3/1 -> Data Type Conversion8/1
  Ground4/1 -> Data Type Conversion9/1
  Ground5/1 -> Data Type Conversion10/1
  Data Type Conversion11/1 -> buscreator/2  "NumOfTarget"
  Bus Selector/2 -> Data Type Conversion11/1  "<VOUTP_NumberOfTargets_num>"

== system hcu_main_ADASwEPS/User2CAN1_/EPAS2 ==
  BOSP_outputs : Inport
  Bus Selector : BusSelector  OutputSignals=VOSP_EPAS2CalcChecksum_raw8,VOSP_EPAS2RollCnt_cnt,VOSP_RelStrAng_deg,VOSP_StrTq_Nm,VOSP_StrTqValid_flg,VOSP_RelStrAngValid_flg,VOSP_EpasFailed_flg,VOSP_ElectPWRConsumpt_A
  Logical Operator : Logic  Operator=NOT  AllPortsSameDT=off  OutDataTypeStr=boolean
  buscreator : BusCreator  Inputs=8
  dt_Elect_PWR_Consumpt : DataTypeConversion  RndMeth=Zero
  dt_EpasFailed : DataTypeConversion  RndMeth=Zero
  dt_RSP_OK : DataTypeConversion  RndMeth=Zero
  dt_R_SAS_Angle : DataTypeConversion  RndMeth=Zero
  dt_SAS_CheckSum2 : DataTypeConversion  RndMeth=Zero
  dt_SAS_MsgCount2 : DataTypeConversion  RndMeth=Zero
  dt_Steering_Torque : DataTypeConversion  RndMeth=Zero
  dt_Steering_Torque_V : DataTypeConversion  RndMeth=Zero
  out : Outport
  wires:
  buscreator/1 -> out/1  "EPAS2"
  dt_SAS_CheckSum2/1 -> buscreator/1  "SAS_CheckSum2"
  dt_SAS_MsgCount2/1 -> buscreator/2  "SAS_MsgCount2"
  dt_R_SAS_Angle/1 -> buscreator/3  "R_SAS_Angle"
  dt_Steering_Torque/1 -> buscreator/4  "Steering_Torque"
  dt_Steering_Torque_V/1 -> buscreator/5  "Steering_Torque_V"
  dt_RSP_OK/1 -> buscreator/6  "RSP_OK"
  dt_EpasFailed/1 -> buscreator/7  "EpasFailed"
  dt_Elect_PWR_Consumpt/1 -> buscreator/8  "Elect_PWR_Consumpt"
  Bus Selector/1 -> dt_SAS_CheckSum2/1  "<VOSP_EPAS2CalcChecksum_raw8>"
  Bus Selector/2 -> dt_SAS_MsgCount2/1  "<VOSP_EPAS2RollCnt_cnt>"
  Bus Selector/3 -> dt_R_SAS_Angle/1  "<VOSP_RelStrAng_deg>"
  Bus Selector/4 -> dt_Steering_Torque/1  "<VOSP_StrTq_Nm>"
  Bus Selector/5 -> Logical Operator/1  "<VOSP_StrTqValid_flg>"
  Bus Selector/6 -> dt_RSP_OK/1  "<VOSP_RelStrAngValid_flg>"
  Bus Selector/7 -> dt_EpasFailed/1  "<VOSP_EpasFailed_flg>"
  Bus Selector/8 -> dt_Elect_PWR_Consumpt/1  "<VOSP_ElectPWRConsumpt_A>"
  BOSP_outputs/1 -> Bus Selector/1
  Logical Operator/1 -> dt_Steering_Torque_V/1

== system hcu_main_ADASwEPS/User2CAN1_/EPAS3 ==
  BOSP_outputs : Inport
  Bus Selector : BusSelector  OutputSignals=VOSP_EPAS3CalcChecksum_raw8,VOSP_EPAS3RollCnt_cnt,VOSP_AckStrTqReqAppl_flg,VOSP_AckStrAngReqAppl_flg,VOSP_EPSLFCStatus_enum,VOSP_EPSBattVolt_V,VOSP_AckStrTqReq_Nm,VOSP_EPSADASAbReason_enum,VOSP_EPSLKAStatus_enum,VOSP_AckStrAngReq_deg
  buscreator : BusCreator  Inputs=10
  dt_SAS_CheckSum{1..10} (10 alike) : DataTypeConversion  RndMeth=Zero
  out : Outport
  wires:
  buscreator/1 -> out/1  "EPAS3"
  dt_SAS_CheckSum2/1 -> buscreator/1  "EPAS3_Checksum"
  dt_SAS_CheckSum1/1 -> buscreator/2  "EPAS3_LifeCount"
  dt_SAS_CheckSum3/1 -> buscreator/3  "CurStrTqReq_A"
  dt_SAS_CheckSum4/1 -> buscreator/4  "CurStrAngReq_A"
  dt_SAS_CheckSum5/1 -> buscreator/5  "EPSLFCStatus"
  dt_SAS_CheckSum6/1 -> buscreator/6  "EPSBattVolt"
  dt_SAS_CheckSum7/1 -> buscreator/7  "CurStrTqReq"
  dt_SAS_CheckSum8/1 -> buscreator/8  "EPSADASAbReason"
  dt_SAS_CheckSum9/1 -> buscreator/9  "EPSLKAStatus"
  dt_SAS_CheckSum10/1 -> buscreator/10  "CurStrAngReq"
  BOSP_outputs/1 -> Bus Selector/1
  Bus Selector/1 -> dt_SAS_CheckSum2/1  "<VOSP_EPAS3CalcChecksum_raw8>"
  Bus Selector/2 -> dt_SAS_CheckSum1/1  "<VOSP_EPAS3RollCnt_cnt>"
  Bus Selector/3 -> dt_SAS_CheckSum3/1  "<VOSP_AckStrTqReqAppl_flg>"
  Bus Selector/4 -> dt_SAS_CheckSum4/1  "<VOSP_AckStrAngReqAppl_flg>"
  Bus Selector/5 -> dt_SAS_CheckSum5/1  "<VOSP_EPSLFCStatus_enum>"
  Bus Selector/6 -> dt_SAS_CheckSum6/1  "<VOSP_EPSBattVolt_V>"
  Bus Selector/7 -> dt_SAS_CheckSum7/1  "<VOSP_AckStrTqReq_Nm>"
  Bus Selector/8 -> dt_SAS_CheckSum8/1  "<VOSP_EPSADASAbReason_enum>"
  Bus Selector/9 -> dt_SAS_CheckSum9/1  "<VOSP_EPSLKAStatus_enum>"
  Bus Selector/10 -> dt_SAS_CheckSum10/1  "<VOSP_AckStrAngReq_deg>"

== system hcu_main_ADASwEPS/User2CAN1_/SAS1 ==
  BOSP_outputs : Inport
  Bus Selector : BusSelector  OutputSignals=VOSP_SAS1CalcChecksum_raw8,VOSP_SAS1RollCnt_cnt,VOSP_StrAngSensorValid_flg,VOSP_StrAngCal_flg,VOSP_StrAng_deg
  buscreator : BusCreator  Inputs=5
  dt_SAS_Angle : DataTypeConversion  RndMeth=Zero
  dt_SAS_CAL : DataTypeConversion  RndMeth=Zero
  dt_SAS_CheckSum : DataTypeConversion  RndMeth=Zero
  dt_SAS_MsgCount : DataTypeConversion  RndMeth=Zero
  dt_SAS_OK : DataTypeConversion  RndMeth=Zero
  out : Outport
  wires:
  buscreator/1 -> out/1  "SAS1"
  dt_SAS_CheckSum/1 -> buscreator/1  "SAS_CheckSum"
  dt_SAS_MsgCount/1 -> buscreator/2  "SAS_MsgCount"
  dt_SAS_OK/1 -> buscreator/3  "SAS_OK"
  dt_SAS_CAL/1 -> buscreator/4  "SAS_CAL"
  dt_SAS_Angle/1 -> buscreator/5  "SAS_Angle"
  Bus Selector/3 -> dt_SAS_OK/1  "<VOSP_StrAngSensorValid_flg>"
  Bus Selector/2 -> dt_SAS_MsgCount/1  "<VOSP_SAS1RollCnt_cnt>"
  Bus Selector/4 -> dt_SAS_CAL/1  "<VOSP_StrAngCal_flg>"
  Bus Selector/1 -> dt_SAS_CheckSum/1  "<VOSP_SAS1CalcChecksum_raw8>"
  Bus Selector/5 -> dt_SAS_Angle/1  "<VOSP_StrAng_deg>"
  BOSP_outputs/1 -> Bus Selector/1

== system hcu_main_ADASwEPS/User2CAN2/ABS2_C ==
  CAN1_Rx1 : Inport
  Bus Selector2 : BusSelector  OutputSignals=ABS2.BrkSw_Sta,ABS2.BrkSw_V,ABS2.VehSpeed
  Data Type Conversion3 : DataTypeConversion
  Data Type Conversion4 : DataTypeConversion
  Data Type Conversion5 : DataTypeConversion
  buscreator : BusCreator  Inputs=3
  out : Outport
  wires:
  buscreator/1 -> out/1  "ABS2_C"
  Data Type Conversion3/1 -> buscreator/1  "BrkSw_Sta"
  Data Type Conversion4/1 -> buscreator/2  "BrkSw_V"
  Data Type Conversion5/1 -> buscreator/3  "VehSpeed"
  Bus Selector2/1 -> Data Type Conversion3/1  "<BrkSw_Sta>"
  Bus Selector2/2 -> Data Type Conversion4/1  "<BrkSw_V>"
  Bus Selector2/3 -> Data Type Conversion5/1  "<VehSpeed>"
  CAN1_Rx1/1 -> Bus Selector2/1

== system hcu_main_ADASwEPS/User2CAN2/ABS4_C ==
  CAN1_Rx : Inport
  Bus Selector1 : BusSelector  OutputSignals=ABS4.YawRate,ABS4.YawRate_V
  Data Type Conversion : DataTypeConversion
  Data Type Conversion3 : DataTypeConversion
  buscreator : BusCreator  Inputs=2
  out : Outport
  wires:
  buscreator/1 -> out/1  "ABS4_C"
  Data Type Conversion/1 -> buscreator/1  "YawRate"
  Data Type Conversion3/1 -> buscreator/2  "YawRate_V"
  CAN1_Rx/1 -> Bus Selector1/1
  Bus Selector1/1 -> Data Type Conversion/1  "<YawRate>"
  Bus Selector1/2 -> Data Type Conversion3/1  "<YawRate_V>"

== system hcu_main_ADASwEPS/User2CAN2/BCM1_C ==
  CAN1_Rx : Inport
  Bus Selector1 : BusSelector  OutputSignals=BCM1.BCM_RTurnLp_Sta,BCM1.BCM_LTurnLp_Sta
  Data Type Conversion : DataTypeConversion
  Data Type Conversion3 : DataTypeConversion
  buscreator : BusCreator  Inputs=2
  out : Outport
  wires:
  buscreator/1 -> out/1  "BCM1_C"
  Data Type Conversion/1 -> buscreator/1  "BCM_RTurnLp_Sta"
  Data Type Conversion3/1 -> buscreator/2  "BCM_LTurnLp_Sta"
  CAN1_Rx/1 -> Bus Selector1/1
  Bus Selector1/1 -> Data Type Conversion/1  "<BCM_RTurnLp_Sta>"
  Bus Selector1/2 -> Data Type Conversion3/1  "<BCM_LTurnLp_Sta>"

== system hcu_main_ADASwEPS/User2CAN2/CSW1_C ==
  CAN1_Rx : Inport
  Bus Selector1 : BusSelector  OutputSignals=CSW1.CSW_FWipSw_Sta
  Data Type Conversion : DataTypeConversion
  buscreator : BusCreator  Inputs=1
  out : Outport
  wires:
  buscreator/1 -> out/1  "CSW1_C"
  Data Type Conversion/1 -> buscreator/1  "CSW_FWipSw_Sta"
  CAN1_Rx/1 -> Bus Selector1/1
  Bus Selector1/1 -> Data Type Conversion/1  "<CSW_FWipSw_Sta>"

== system hcu_main_ADASwEPS/User2CAN2/FECU1_C ==
  CAN1_Rx : Inport
  Bus Selector1 : BusSelector  OutputSignals=FECU1.FECU_HiBeamRly_Sta
  Data Type Conversion : DataTypeConversion
  buscreator : BusCreator  Inputs=1
  out : Outport
  wires:
  buscreator/1 -> out/1  "FECU1_C"
  Data Type Conversion/1 -> buscreator/1  "FECU_HiBeamRly_Sta"
  CAN1_Rx/1 -> Bus Selector1/1
  Bus Selector1/1 -> Data Type Conversion/1  "<FECU_HiBeamRly_Sta>"

== system hcu_main_ADASwEPS/User2CAN2/SAS1_C ==
  CAN1_Rx : Inport
  Bus Selector1 : BusSelector  OutputSignals=SAS1.SAS_OK,SAS1.SAS_CAL,SAS1.SAS_Angle
  Data Type Conversion3 : DataTypeConversion
  Data Type Conversion4 : DataTypeConversion
  Data Type Conversion5 : DataTypeConversion
  buscreator : BusCreator  Inputs=3
  out : Outport
  wires:
  buscreator/1 -> out/1  "SAS1_C"
  Data Type Conversion3/1 -> buscreator/1  "SAS_OK"
  Data Type Conversion4/1 -> buscreator/2  "SAS_CAL"
  Data Type Conversion5/1 -> buscreator/3  "SAS_Angle"
  CAN1_Rx/1 -> Bus Selector1/1
  Bus Selector1/1 -> Data Type Conversion3/1  "<SAS_OK>"
  Bus Selector1/2 -> Data Type Conversion4/1  "<SAS_CAL>"
  Bus Selector1/3 -> Data Type Conversion5/1  "<SAS_Angle>"

== system hcu_main_ADASwEPS/User2CAN2/SpeedInformation ==
  CAN1_Rx : Inport
  Bus Selector1 : BusSelector  OutputSignals=ABS2.VehSpeed
  Bus Selector2 : BusSelector  OutputSignals=TCM1.CAN_GEAR_STATE_NOW
  Constant : Constant  Value=single(0)
  Constant1 : Constant  Value=uint8(0)
  Constant10 : Constant  Value=uint8(2)
  Constant11 : Constant  Value=uint8(3)
  Constant2 : Constant  Value=ENUM_GEARPOSN_1ST
  Constant3 : Constant  Value=ENUM_GEARPOSN_2ND
  Constant4 : Constant  Value=ENUM_GEARPOSN_3RD
  Constant5 : Constant  Value=ENUM_GEARPOSN_4TH
  Constant6 : Constant  Value=ENUM_GEARPOSN_5TH
  Constant7 : Constant  Value=ENUM_GEARPOSN_6TH
  Constant8 : Constant  Value=ENUM_GEARPOSN_R
  Constant9 : Constant  Value=uint8(1)
  Data Type Conversion1 : DataTypeConversion
  Data Type Conversion2 : DataTypeConversion
  Gain : Gain  Gain=1000/3600
  Logical Operator : Logic  Operator=OR  Inputs=6  AllPortsSameDT=off  OutDataTypeStr=boolean
  Relational Operator{,1..7} (8 alike) : RelationalOperator  Operator===  OutDataTypeStr=boolean
  Switch : Switch  Criteria=u2 ~= 0
  Switch1 : Switch  Criteria=u2 ~= 0
  Switch2 : Switch  Criteria=u2 ~= 0
  buscreator : BusCreator  Inputs=2
  out : Outport
  wires:
  buscreator/1 -> out/1  "SpeedInformation"
  Data Type Conversion2/1 -> buscreator/2  "radarDeviceSpeedDirection"
  Data Type Conversion1/1 -> buscreator/1  "radarDeviceSpeed"
  CAN1_Rx/1 -> Bus Selector2/1, Bus Selector1/1
  Bus Selector1/1 -> Relational Operator/1, Gain/1  "<VehSpeed>"
  Bus Selector2/1 -> Relational Operator3/1, Relational Operator4/1, Relational Operator5/1, Relational Operator6/1, Relational Operator7/1, Relational Operator2/1, Relational Operator1/1  "<CAN_GEAR_STATE_NOW>"
  Gain/1 -> Data Type Conversion1/1
  Switch/1 -> Data Type Conversion2/1
  Relational Operator/1 -> Switch/2
  Constant/1 -> Relational Operator/2
  Constant1/1 -> Switch/1
  Constant2/1 -> Relational Operator1/2
  Constant3/1 -> Relational Operator2/2
  Constant4/1 -> Relational Operator3/2
  Constant5/1 -> Relational Operator4/2
  Constant6/1 -> Relational Operator5/2
  Constant7/1 -> Relational Operator6/2
  Constant8/1 -> Relational Operator7/2
  Relational Operator1/1 -> Logical Operator/1
  Relational Operator2/1 -> Logical Operator/2
  Relational Operator3/1 -> Logical Operator/3
  Relational Operator4/1 -> Logical Operator/4
  Relational Operator5/1 -> Logical Operator/5
  Relational Operator6/1 -> Logical Operator/6
  Switch1/1 -> Switch/3
  Logical Operator/1 -> Switch1/2
  Constant9/1 -> Switch1/1
  Switch2/1 -> Switch1/3
  Relational Operator7/1 -> Switch2/2
  Constant10/1 -> Switch2/1
  Constant11/1 -> Switch2/3

== system hcu_main_ADASwEPS/User2CAN2/YawRateInformation ==
  CAN1_Rx : Inport
  Bus Selector1 : BusSelector  OutputSignals=ABS4.YawRate
  Data Type Conversion1 : DataTypeConversion
  Gain : Gain  Gain=-1
  buscreator : BusCreator  Inputs=1
  out : Outport
  wires:
  buscreator/1 -> out/1  "YawRateInformation"
  Data Type Conversion1/1 -> buscreator/1  "radarDeviceYawRate"
  CAN1_Rx/1 -> Bus Selector1/1
  Bus Selector1/1 -> Gain/1  "<YawRate>"
  Gain/1 -> Data Type Conversion1/1
